simulink model "CarOpenLoop"  (Simulink 7.7)
settings: Solver=ode45  StartTime=0.0  StopTime=10.0  RelTol=1e-3
values from neighbouring files (symbols this model uses):
  L = 0.2    [car1.m]    (also in car2.m; car3.m; car4.m)
libraries: simulink x1
settings Model: Creator=mauricio  LastModifiedBy=mauricio

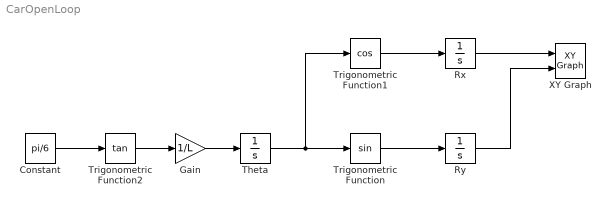
== system CarOpenLoop ==
  Constant : Constant  Value=pi/6
  Gain : Gain  Gain=1/L
  Rx : Integrator
  Ry : Integrator
  Theta : Integrator
  Trigonometric Function : Trigonometry
  Trigonometric Function1 : Trigonometry  Operator=cos
  Trigonometric Function2 : Trigonometry  Operator=tan
  XY Graph : simulink/Sinks/XY Graph  SystemSampleTime=-1  xmin=-1  xmax=1  ymin=-1  ymax=1  st=-1
  wires:
  Trigonometric Function1/1 -> Rx/1
  Trigonometric Function/1 -> Ry/1
  Theta/1 -> Trigonometric Function/1, Trigonometric Function1/1
  Trigonometric Function2/1 -> Gain/1
  Gain/1 -> Theta/1
  Constant/1 -> Trigonometric Function2/1
  Rx/1 -> XY Graph/1
  Ry/1 -> XY Graph/2
